simulink model "AAI"  (R2022a)
settings: Solver=FixedStepAuto  StartTime=0.0  StopTime=10.0  FixedStep=1e-3  RelTol=1e-3  EnableMultiTasking=on
undefined symbols (not defined in the file): D0, D10, D11, D12, D13, D2, D3, D4, D5, D6, D7, D8, D9, PTA0, PTA1, PTA2, PTB23, PTB9, PTC16, PTC2, PTC3, PTC4, PTD0, PTD1, PTD2, PTD3
libraries: frdmk64flib x14
settings Model: ExtModeTrigDuration=5  Creator=12791  LastModifiedBy=12791
settings OptimizationCC: EnhancedBackFolding=on  PassReuseOutputArgsAs=Individual arguments  ZeroExternalMemoryAtStartup=off  ZeroInternalMemoryAtStartup=off  MaxStackSize=64  OptimizeBlockOrder=speed  DifferentSizesBufferReuse=on  OptimizationCustomize=off  EfficientTunableParamExpr=on
settings DebuggingCC: ParameterTunabilityLossMsg=error
settings HardwareCC: ProdBitPerPointer=32  ProdBitPerSizeT=32  ProdBitPerPtrDiffT=32  ProdLargestAtomicInteger=Long  ProdLargestAtomicFloat=Double  ProdWordSize=32  ProdHWDeviceType=ARM Compatible->ARM Cortex
settings SFSimCC: MATLABDynamicMemAlloc=off
settings RTWCC: SystemTargetFile=ert.tlc  HardwareBoard=NXP FRDM-K64F  TLCOptions="-aInlineSetEventsForThisBaseRateFcn=TLC_FALSE -aSuppressMultiTaskScheduler=TLC_FALSE  -aRateBasedStepFcn=0"  TemplateMakefile=ert_default_tmf  Toolchain=GNU Tools for ARM Embedded Processors
settings CodeAppCC: ForceParamTrailComments=on  IgnoreCustomStorageClasses=off  OperatorAnnotations=on  SimulinkDataObjDesc=on  SFDataObjDesc=on  InsertBlockDesc=on
settings ERTTargetCC: ExtModeTransport=4  ExtModeMexFile=sendToCommService

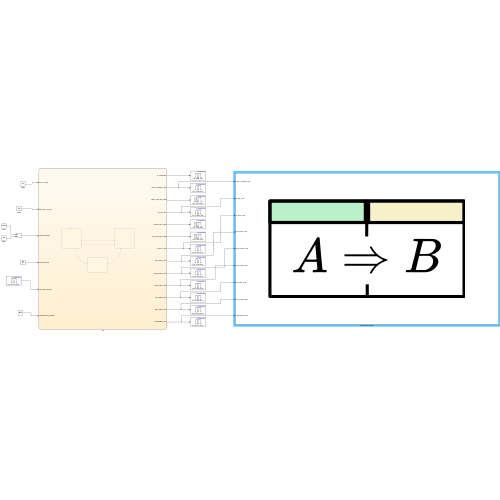
[thumbnail: Simulink's stored preview of the top-level diagram]
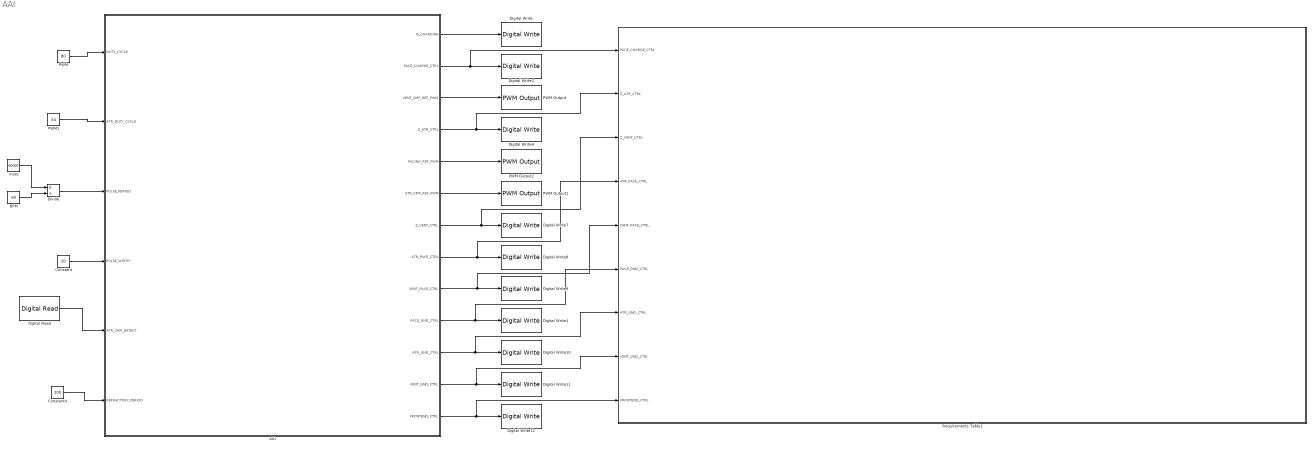
== system AAI ==
  AAI : Stateflow chart  TreatAsAtomicUnit=on
  BPM : Constant  Value=60
  Constant : Constant  Value=20
  Constant4 : Constant  Value=200
  Digital Read : frdmk64flib/Digital Read  Whichpin=PTC16 (D0)  SampleTime=-1
  Digital Write : frdmk64flib/Digital Write  Whichpin=RED_LED
  Digital Write1 : frdmk64flib/Digital Write  Whichpin=PTD0 (D10)
  Digital Write10 : frdmk64flib/Digital Write  Whichpin=PTD2 (D11)
  Digital Write11 : frdmk64flib/Digital Write  Whichpin=PTD3 (D12)
  Digital Write12 : frdmk64flib/Digital Write  Whichpin=PTD1 (D13)
  Digital Write2 : frdmk64flib/Digital Write  Whichpin=PTB9 (D2)
  Digital Write4 : frdmk64flib/Digital Write  Whichpin=PTB23 (D4)
  Digital Write7 : frdmk64flib/Digital Write  Whichpin=PTC3 (D7)
  Digital Write8 : frdmk64flib/Digital Write  Whichpin=PTA0 (D8)
  Digital Write9 : frdmk64flib/Digital Write  Whichpin=PTC4 (D9)
  Divide : Product  Inputs=*/
  PWM : Constant  Value=80
  PWM Output : frdmk64flib/PWM Output  Whichpin=PTA1 (D3)  InitialFrequency=2000  InitialDutyCycle=0
  PWM Output1 : frdmk64flib/PWM Output  Whichpin=PTC2 (D6)  InitialFrequency=2000  InitialDutyCycle=0
  PWM Output2 : frdmk64flib/PWM Output  Whichpin=PTA2 (D5)  InitialFrequency=2000  InitialDutyCycle=0
  PWM1 : Constant  Value=54
  Requirements Table1 : Requirements Table  TreatAsAtomicUnit=on
  msec : Constant  Value=60000
  wires:
  AAI/2(PACE_CHARGE_CTRL) -> Requirements Table1/1(PACE_CHARGE_CTRL), Digital Write2/1
  AAI/7(Z_VENT_CTRL) -> Requirements Table1/3(Z_VENT_CTRL), Digital Write7/1
  AAI/9(VENT_PACE_CTRL) -> Requirements Table1/5(VENT_PACE_CTRL), Digital Write9/1
  AAI/10(PACE_GND_CTRL) -> Requirements Table1/6(PACE_GND_CTRL), Digital Write1/1
  AAI/11(ATR_GND_CTRL) -> Requirements Table1/7(ATR_GND_CTRL), Digital Write10/1
  AAI/12(VENT_GND_CTRL) -> Requirements Table1/8(VENT_GND_CTRL), Digital Write11/1
  AAI/13(FRONTEND_CTRL) -> Requirements Table1/9(FRONTEND_CTRL), Digital Write12/1
  PWM/1 -> AAI/1(DUTY_CYCLE)
  Constant/1 -> AAI/4(PULSE_WIDTH)
  Divide/1 -> AAI/3(PULSE_PERIOD)
  msec/1 -> Divide/1
  BPM/1 -> Divide/2
  AAI/1(IS_CHARGING) -> Digital Write/1
  AAI/5(PACING_REF_PWM) -> PWM Output2/1
  Digital Read/1 -> AAI/5(ATR_CMP_DETECT)
  Constant4/1 -> AAI/6(REFRACTORY_PERIOD)
  AAI/3(VENT_CMP_REF_PWM) -> PWM Output/1
  AAI/6(ATR_CMP_REF_PWM) -> PWM Output1/1
  PWM1/1 -> AAI/2(ATR_DUTY_CYCLE)
  AAI/4(Z_ATR_CTRL) -> Requirements Table1/2(Z_ATR_CTRL), Digital Write4/1
  AAI/8(ATR_PACE_CTRL) -> Requirements Table1/4(ATR_PACE_CTRL), Digital Write8/1

== stateflow chart AAI/Requirements Table1 ==
  (default) -> (junction 1073743086)
  (junction 1073743086) -> (junction 1073743087) : {
      | % SF_REQ_REV_07
      | }
  (junction 1073743087) -> (junction 1073743089) : {
      | % HEADER_ASSIGNMENTS
      |
      | }
  (junction 1073743089) -> (junction 1073743091) : {
      | % START_A_4
      | }
  (junction 1073743091) -> (junction 1073743093) : {
      | }
  (junction 1073743093) -> (junction 1073743095)
  (junction 1073743095) -> (junction 1073743097) : {
      | }
  (junction 1073743097) -> (junction 1073743099) : {
      | % END_A_4
      | }
  (junction 1073743099) -> (junction 1073743101) : {
      | % START_R_1
      | }
  (junction 1073743101) -> (junction 1073743103) : {
      | }
  (junction 1073743103) -> (junction 1073743105) : {
      |
      |
      | }
  (junction 1073743105) -> (junction 1073743107) : {
      | }
  (junction 1073743107) -> (junction 1073743109) : {
      | % START_R_7
      | }
  (junction 1073743109) -> (junction 1073743111) : {
      | }
  (junction 1073743111) -> (junction 1073743113)
  (junction 1073743113) -> (junction 1073743115) [order 1] : [(((prev(PACE_CHARGE_CTRL)) == (1))) && (((prev(Z_ATR_CTRL)) == (0))) && (((prev(Z_VENT_CTRL)) == (0))) && (((prev(ATR_PACE_CTRL)) == (0))) && (((prev(VENT_PACE_CTRL)) == (0))) && (((prev(PACE_GND_CTRL)) == (1))) && (((prev(ATR_GND_CTRL)) == (1))) && (((prev(VENT_GND_CTRL)) == (0))) && (((prev(FRONTEND_CTRL)) == (1)))]
  (junction 1073743113) -> (junction 1073743121) [order 2]
  (junction 1073743115) -> (junction 1073743117) : {
      | reqtable_postcondition((((PACE_CHARGE_CTRL) == (1))) && (((Z_ATR_CTRL) == (0))) && (((Z_VENT_CTRL) == (0))) && (((ATR_PACE_CTRL) == (0))) && (((VENT_PACE_CTRL) == (0))) && (((PACE_GND_CTRL) == (1))) && (((ATR_GND_CTRL) == (1))) && (((VENT_GND_CTRL) == (0))) && (((FRONTEND_CTRL) == (1))), 'R:1.1');
      |
      |
      | }
  (junction 1073743117) -> (junction 1073743119) : {
      | }
  (junction 1073743119) -> (junction 1073743121)
  (junction 1073743121) -> (junction 1073743123)
  (junction 1073743123) -> (junction 1073743125) : {
      | % END_R_7
      | }
  (junction 1073743125) -> (junction 1073743170) : {
      | % START_R_13
      | }
  (junction 1073743170) -> (junction 1073743172) : {
      | }
  (junction 1073743172) -> (junction 1073743174)
  (junction 1073743174) -> (junction 1073743176) [order 1] : [(((prev(PACE_CHARGE_CTRL)) == (1))) && (((prev(Z_ATR_CTRL)) == (0))) && (((prev(Z_VENT_CTRL)) == (0))) && (((prev(ATR_PACE_CTRL)) == (0))) && (((prev(VENT_PACE_CTRL)) == (0))) && (((prev(PACE_GND_CTRL)) == (1))) && (((prev(ATR_GND_CTRL)) == (1))) && (((prev(VENT_GND_CTRL)) == (0))) && (((prev(FRONTEND_CTRL)) == (1)))]
  (junction 1073743174) -> (junction 1073743182) [order 2]
  (junction 1073743176) -> (junction 1073743178) : {
      | reqtable_postcondition((((PACE_CHARGE_CTRL) == (1))) && (((Z_ATR_CTRL) == (0))) && (((Z_VENT_CTRL) == (0))) && (((ATR_PACE_CTRL) == (0))) && (((VENT_PACE_CTRL) == (0))) && (((PACE_GND_CTRL) == (1))) && (((ATR_GND_CTRL) == (1))) && (((VENT_GND_CTRL) == (0))) && (((FRONTEND_CTRL) == (1))), 'R:1.2');
      |
      |
      | }
  (junction 1073743178) -> (junction 1073743180) : {
      | }
  (junction 1073743180) -> (junction 1073743182)
  (junction 1073743182) -> (junction 1073743184)
  (junction 1073743184) -> (junction 1073743186) : {
      | % END_R_13
      | }
  (junction 1073743186) -> (junction 1073743127) : {
      | % START_R_10
      | }
  (junction 1073743127) -> (junction 1073743129) : {
      | }
  (junction 1073743129) -> (junction 1073743131)
  (junction 1073743131) -> (junction 1073743133) [order 1] : [(((prev(PACE_CHARGE_CTRL)) == (0))) && (((prev(Z_ATR_CTRL)) == (0))) && (((prev(Z_VENT_CTRL)) == (0))) && (((prev(ATR_PACE_CTRL)) == (1))) && (((prev(VENT_PACE_CTRL)) == (0))) && (((prev(PACE_GND_CTRL)) == (1))) && (((prev(ATR_GND_CTRL)) == (0))) && (((prev(VENT_GND_CTRL)) == (0))) && (((prev(FRONTEND_CTRL)) == (1)))]
  (junction 1073743131) -> (junction 1073743139) [order 2]
  (junction 1073743133) -> (junction 1073743135) : {
      | reqtable_postcondition((((PACE_CHARGE_CTRL) == (0))) && (((Z_ATR_CTRL) == (0))) && (((Z_VENT_CTRL) == (0))) && (((ATR_PACE_CTRL) == (1))) && (((VENT_PACE_CTRL) == (0))) && (((PACE_GND_CTRL) == (1))) && (((ATR_GND_CTRL) == (0))) && (((VENT_GND_CTRL) == (0))) && (((FRONTEND_CTRL) == (1))), 'R:1.3');
      |
      |
      | }
  (junction 1073743135) -> (junction 1073743137) : {
      | }
  (junction 1073743137) -> (junction 1073743139)
  (junction 1073743139) -> (junction 1073743141)
  (junction 1073743141) -> (junction 1073743161) : {
      | % END_R_10
      | }
  (junction 1073743161) -> (junction 1073743163) : {
      | % END_R_1
      | }
  data: PACE_CHARGE_CTRL input boolean; Z_ATR_CTRL input boolean; Z_VENT_CTRL input boolean; ATR_PACE_CTRL input boolean; VENT_PACE_CTRL input boolean; PACE_GND_CTRL input boolean; ATR_GND_CTRL input boolean; VENT_GND_CTRL input boolean; FRONTEND_CTRL input boolean =true

== stateflow chart AAI/AAI ==
  state Charging_C22
    entry:
    PACING_REF_PWM = DUTY_CYCLE
    PACE_CHARGE_CTRL = true
    PACE_GND_CTRL = true
    ATR_PACE_CTRL = false
    Z_ATR_CTRL = false
    Z_VENT_CTRL = false
    VENT_PACE_CTRL = false
    VENT_GND_CTRL = false
    ATR_GND_CTRL = true
    % For LED testing
    IS_CHARGING = true
    ATR_CMP_REF_PWM = ATR_DUTY_CYCLE
    FRONTEND_CTRL = true
  state Proxy
    entry:
    PACING_REF_PWM = DUTY_CYCLE
    PACE_CHARGE_CTRL = true
    PACE_GND_CTRL = true
    ATR_PACE_CTRL = false
    Z_ATR_CTRL = false
    Z_VENT_CTRL = false
    VENT_PACE_CTRL = false
    VENT_GND_CTRL = false
    ATR_GND_CTRL = true
    % For LED testing
    IS_CHARGING = true
    ATR_CMP_REF_PWM = ATR_DUTY_CYCLE
  state Pacing
    entry:
    PACE_CHARGE_CTRL = false
    PACE_GND_CTRL = true
    VENT_PACE_CTRL = false
    VENT_GND_CTRL = false
    Z_ATR_CTRL = false
    Z_VENT_CTRL = false
    ATR_GND_CTRL = false
    ATR_PACE_CTRL = true
    % For LED testing
    IS_CHARGING = false
  (default) -> Charging_C22
  Charging_C22 -> Proxy [order 1] : [ATR_CMP_DETECT ==  true]{DELAY = REFRACTORY_PERIOD}
  Proxy -> Charging_C22 : [after(DELAY,msec)]
  Charging_C22 -> Pacing [order 2] : [after(PULSE_PERIOD-REFRACTORY_PERIOD,msec)]
  Pacing -> Proxy : [after(PULSE_WIDTH,msec)]{DELAY = REFRACTORY_PERIOD - PULSE_WIDTH }
  data: IS_CHARGING output; PACE_CHARGE_CTRL output; VENT_CMP_REF_PWM output =0; Z_ATR_CTRL output; PACING_REF_PWM output; ATR_CMP_REF_PWM output =0; Z_VENT_CTRL output; ATR_PACE_CTRL output; VENT_PACE_CTRL output; PACE_GND_CTRL output; ATR_GND_CTRL output; VENT_GND_CTRL output; FRONTEND_CTRL output =true; DUTY_CYCLE input; ATR_DUTY_CYCLE input; PULSE_PERIOD input; PULSE_WIDTH input; ATR_CMP_DETECT input; DELAY local; REFRACTORY_PERIOD input
